simulink model "UAV_Research_Environment"  (R2025a)
settings: Solver=ode23t  StartTime=0.0  StopTime=130  MaxStep=2e-3  RelTol=1e-4  AbsTol=1e-3  EnableMultiTasking=on
InitFcn:
  | skipInitialization = false;
  | 
  | if evalin('base', ...
  |         'exist(''CONTROLLER_TUNING_ACTIVE'',''var'')')
  | 
  |     skipInitialization = evalin('base', ...
  |         'logical(CONTROLLER_TUNING_ACTIVE)');
  | end
  | 
  | if ~skipInitialization
  | 
  |     icraControllerPrepared = false;
  | 
  |     hasICRAVariables = evalin('base', ...
  |         ['exist(''AUTOPILOT'',''var'') && ' ...
  |          'exist(''ICRA_ACTIVE_CONTROLLER'',''var'') && ' ...
  |          'exist(''ICRA_ACTIVE_RUN_ID'',''var'')']);
  | 
  |     if hasICRAVariables
  | 
  |         icraControllerPrepared = evalin('base', ...
  |             ['isstruct(AUTOPILOT) && ' ...
  |              'isfield(AUTOPILOT,''info'') && ' ...
  |              'isfield(AUTOPILOT.info,''ICRAControllerID'') && ' ...
  |              'strcmp(string(AUTOPILOT.info.ICRAControllerID), ' ...
  |                     'string(ICRA_ACTIVE_CONTROLLER))']);
  | 
  |     end
  | 
  |     if icraControllerPrepared
  |         skipInitialization = true;
  |     end
  | end
  | 
  | if ~skipInitialization
  | 
  |     mdl = bdroot;
  | 
  |     mdl_file = get_param(mdl, 'FileName');
  | 
  |     project_root = fileparts(mdl_file);
  | 
  |     init_file = fullfile(project_root, 'initialize_project.m');
  | 
  |     if exist(init_file, 'file')
  | 
  |         run(init_file);
  | 
  |     else
  | 
  |         error('initialize_project.m was not found in the model folder.');
  | 
  |     end
  | end
values from neighbouring files (symbols this model uses):
  A_UAV = struct()    [UAV_analytical.m]
  AUTOPILOT = struct()    [UAV_autopilot.m]
  B_UAV = struct()    [UAV_block.m]
  D = A_UAV.source.propeller_diameter_m    [UAV_analytical.m]    (also in plot_controller_results.m = permute(                  D,                  order); plot_estimator_results.m = permute(              D,              order); plot_mission_results.m = permute(                  D,                  order); plot_touchdown_diagnostics.m = permute(                  D,                  order))
  OPERATOR_MODE = OPERATOR_MODE_MANUAL    [initialize_project.m]    (also in uav_remote_gui.m = uint8(0))
  P_ENV = struct()    [Environment.m]
  P_UAV = struct()    [UAV_simscape.m]
  s = sin(angle)    [uav_remote_gui.m]
  SENSOR = struct()    [UAV_sensors.m]
  TRAJECTORY_CONFIG = struct()    [UAV_trajectories.m]
  TRAJECTORY_ID = uint8(          trajectoryIDNumeric)    [UAV_trajectories.m]
  X = reshape(                  D,                  nt,                  [])    [plot_controller_results.m]    (also in plot_estimator_results.m = reshape(              D,              nt,              []); plot_mission_results.m; plot_touchdown_diagnostics.m; plot_trajectory_3d.m)
  Y = absolutePlanNED(1,:)    [plot_trajectory_3d.m]    (also in uav_remote_gui.m = positionNED(:,1))
  Z = landedCGDown -          absolutePlanNED(3,:)    [plot_trajectory_3d.m]    (also in uav_remote_gui.m = landedCGDown-positionNED(:,3))
undefined symbols (not defined in the file or in its folder): Acceleration_ref, F, fractalcoef, Light, MIL, Position_ref, Velocity_ref, Yaw_ref, YawRate_ref
libraries: sm_lib x49, nesl_utility x29, fl_lib x17, slpidlib x16, simulink x14, ee_lib x5, sdl_lib x4, aerolibwind2 x3, aerolibatmos2 x2, sensorbarometerlib x1, sensorgpslib x1, mspsensorlib x1
(part 2 of 9)

== system UAV_Research_Environment/Remote Controller/Automatic Operator ==
  Automatic Protocol : MATLAB Function  TreatAsAtomicUnit=on
  Protocol Table : Constant  Value=|  OutDataTypeStr=double
      | [AUTO_PROTOCOL.selected.armTime_s;
      |  AUTO_PROTOCOL.selected.runTime_s;
      |  AUTO_PROTOCOL.selected.disarmTime_s;
      |  AUTO_PROTOCOL.selected.stopTime_s]
  Simulation Time : Clock
  Trajectory ID : Constant  Value=TRAJECTORY_ID  OutDataTypeStr=uint8
  ArmCommand : Outport
  RunTrajectoryRequestID : Outport  Port=2
  wires:
  Simulation Time/1 -> Automatic Protocol/1(t)
  Trajectory ID/1 -> Automatic Protocol/2(TrajectoryID)
  Protocol Table/1 -> Automatic Protocol/3(ProtocolTable_s)
  Automatic Protocol/1(ArmCommand) -> ArmCommand/1
  Automatic Protocol/2(RunTrajectoryRequestID) -> RunTrajectoryRequestID/1

== system UAV_Research_Environment/Sensor/Barometer ==
  Env : Inport
  Barometer Sensor : sensorbarometerlib/Barometer  ConstantBias=SENSOR.Barometer.constantBias_Pa  NoiseDensity=SENSOR.Barometer.noiseDensity_Pa_sqrtHz  BiasInstability=SENSOR.Barometer.biasInstability_Pa  DecayFactor=SENSOR.Barometer.decayFactor  SeedDouble=SENSOR.Barometer.seed  SimulateUsing=Code generation
      settings: LibrarySourceBlock=uavsimlib/Barometer
  Bus Creator : BusCreator  Inputs=2
  Bus Selector : BusSelector  OutputSignals=Atmosphere.AirPressure
  Pressure Altitude Sensor : aerolibatmos2/Pressure Altitude  units=Metric (MKS)  action=Warning
  Zero-Order Hold : ZeroOrderHold  SampleTime=SENSOR.Barometer.sampleTime_s
  Barometer : Outport
  wires:
  Env/1 -> Bus Selector/1
  Bus Selector/1 -> Zero-Order Hold/1  "<AirPressure>"
  Zero-Order Hold/1 -> Barometer Sensor/1
  Barometer Sensor/1 -> Pressure Altitude Sensor/1, Bus Creator/1  "Pressure"
  Pressure Altitude Sensor/1 -> Bus Creator/2  "Altitude"
  Bus Creator/1 -> Barometer/1

== system UAV_Research_Environment/Sensor/GPS ==
  States : Inport
  Bus Creator : BusCreator  Inputs=2
  Bus Selector : BusSelector  OutputSignals=Position,Velocity
  GPS Sensor : sensorgpslib/GPS  DispRefFrame=NED  PositionInputFormat=Local  ReferenceLocation=SENSOR.GPS.referenceLocation_lla_deg_m  HorizontalPositionAccuracy=SENSOR.GPS.horizontalPositionAccuracy_m  VerticalPositionAccuracy=SENSOR.GPS.verticalPositionAccuracy_m  VelocityAccuracy=SENSOR.GPS.velocityAccuracy_m_s  DecayFactor=SENSOR.GPS.decayFactor  SeedDouble=SENSOR.GPS.seed  SimulateUsing=Code generation
      settings: LibrarySourceBlock=mspsensorlib/GPS
  Reshape : Reshape  OutputDimensionality=Row vector (2-D)
  Reshape1 : Reshape  OutputDimensionality=Row vector (2-D)
  Terminator : Terminator
  Terminator1 : Terminator
  Transpose2 : Math  Operator=transpose
  Transpose3 : Math  Operator=transpose
  Zero-Order Hold : ZeroOrderHold  SampleTime=SENSOR.GPS.sampleTime_s
  Zero-Order Hold1 : ZeroOrderHold  SampleTime=SENSOR.GPS.sampleTime_s
  GPS : Outport
  wires:
  States/1 -> Bus Selector/1
  Bus Selector/1 -> Zero-Order Hold/1  "<Position>"
  Bus Selector/2 -> Zero-Order Hold1/1  "<Velocity>"
  Zero-Order Hold1/1 -> Reshape1/1
  Zero-Order Hold/1 -> Reshape/1
  GPS Sensor/1 -> Transpose2/1  "LLA"
  GPS Sensor/2 -> Transpose3/1  "Velocity"
  Bus Creator/1 -> GPS/1
  Reshape/1 -> GPS Sensor/1
  Reshape1/1 -> GPS Sensor/2
  Transpose2/1 -> Bus Creator/1  "LLA"
  Transpose3/1 -> Bus Creator/2  "Velocity"
  GPS Sensor/3 -> Terminator/1
  GPS Sensor/4 -> Terminator1/1

== system UAV_Research_Environment/Sensor/IMU ==
  States : Inport
  Bus Creator : BusCreator  Inputs=2
  Bus Selector : BusSelector  OutputSignals=Acceleration,AngularRate,Attitude.Q
  IMU Sensor : mspsensorlib/IMU  DispRefFrame=NED  TemperaturePort=off  Temperature=SENSOR.IMU.temperature_C  MagneticFieldPort=off  MagneticFieldNED=SENSOR.IMU.mag.fieldNED_uT  MagneticFieldENU=[ -2.4169, 27.5550, 16.0849 ]  SeedDouble=SENSOR.IMU.seed  SimulateUsing=Code generation  AccelParamsMeasurementRange=SENSOR.IMU.accel.maximumReading_m_s2  AccelParamsResolution=SENSOR.IMU.accel.resolution_m_s2_LSB  AccelParamsConstantBias=SENSOR.IMU.accel.constantBias_m_s2  AccelParamsAxesMisalignment=SENSOR.IMU.accel.axesSkew_percent  AccelParamsNoiseDensity=SENSOR.IMU.accel.velocityRandomWalk_m_s2_sqrtHz  AccelParamsBiasInstability=SENSOR.IMU.accel.biasInstability_m_s2  AccelParamsBiasInstabilityNumerator=fractalcoef().Numerator  AccelParamsBiasInstabilityDenominator=fractalcoef().Denominator  AccelParamsRandomWalk=SENSOR.IMU.accel.accelerationRandomWalk_m_s2_sqrtHz  AccelParamsNoiseType=double-sided  AccelParamsTemperatureBias=[ 0, 0, 0 ]  AccelParamsTemperatureScaleFactor=[ 0, 0, 0 ]  GyroParamsMeasurementRange=SENSOR.IMU.gyro.maximumReading_rad_s  GyroParamsResolution=SENSOR.IMU.gyro.resolution_rad_s_LSB  GyroParamsConstantBias=SENSOR.IMU.gyro.constantBias_rad_s  GyroParamsAxesMisalignment=SENSOR.IMU.gyro.axesSkew_percent  GyroParamsAccelerationBias=SENSOR.IMU.gyro.biasFromAcceleration_rad_s_per_m_s2  GyroParamsNoiseDensity=SENSOR.IMU.gyro.angleRandomWalk_rad_s_sqrtHz  GyroParamsBiasInstability=SENSOR.IMU.gyro.biasInstability_rad_s  GyroParamsBiasInstabilityNumerator=fractalcoef().Numerator  GyroParamsBiasInstabilityDenominator=fractalcoef().Denominator  GyroParamsRandomWalk=SENSOR.IMU.gyro.rateRandomWalk_rad_s_sqrtHz  GyroParamsNoiseType=double-sided  GyroParamsTemperatureBias=SENSOR.IMU.gyro.temperatureBias_rad_s_per_C  GyroParamsTemperatureScaleFactor=SENSOR.IMU.gyro.temperatureScaleFactor_percent_per_C  MagParamsMeasurementRange=SENSOR.IMU.mag.maximumReading_uT  MagParamsResolution=SENSOR.IMU.mag.resolution_uT_LSB  MagParamsConstantBias=SENSOR.IMU.mag.constantBias_uT  MagParamsAxesMisalignment=SENSOR.IMU.mag.axesSkew_percent  MagParamsNoiseDensity=SENSOR.IMU.mag.whiteNoisePSD_uT_sqrtHz  MagParamsBiasInstability=SENSOR.IMU.mag.biasInstability_uT  MagParamsBiasInstabilityNumerator=fractalcoef().Numerator  MagParamsBiasInstabilityDenominator=fractalcoef().Denominator  MagParamsRandomWalk=SENSOR.IMU.mag.randomWalk_uT_sqrtHz  MagParamsNoiseType=double-sided  MagParamsTemperatureBias=SENSOR.IMU.mag.temperatureBias_uT_per_C  MagParamsTemperatureScaleFactor=SENSOR.IMU.mag.temperatureScaleFactor_percent_per_C
  Matrix Multiply : Product  Multiplication=Matrix(*)
  Quaternions to Direction Cosine Matrix : Quat2Dcm
  Reshape : Reshape  OutputDimensionality=Row vector (2-D)
  Reshape2 : Reshape  OutputDimensionality=Customize  OutputDimensions=[3 1]
  Transpose{,1,4..6} (5 alike) : Math  Operator=transpose
  Zero-Order Hold{,1..3} (4 alike) : ZeroOrderHold  SampleTime=SENSOR.IMU.sampleTime_s
  IMU : Outport
  MagneticField : Outport  Port=2
  wires:
  States/1 -> Bus Selector/1
  Bus Selector/1 -> Zero-Order Hold/1  "<Acceleration>"
  Bus Selector/3 -> Quaternions to Direction Cosine Matrix/1  "<Q>"
  Quaternions to Direction Cosine Matrix/1 -> Transpose/1, Zero-Order Hold2/1
  Bus Selector/2 -> Zero-Order Hold3/1  "<AngularRate>"
  Matrix Multiply/1 -> Zero-Order Hold1/1  "Omega_ned"
  IMU Sensor/1 -> Transpose4/1  "Accel"
  IMU Sensor/2 -> Transpose5/1  "Gyro"
  Bus Creator/1 -> IMU/1
  Zero-Order Hold/1 -> Reshape/1
  IMU Sensor/3 -> Transpose6/1
  Reshape/1 -> IMU Sensor/1
  Zero-Order Hold1/1 -> Transpose1/1
  Transpose4/1 -> Bus Creator/1  "Accel"
  Transpose5/1 -> Bus Creator/2  "Gyro"
  Transpose6/1 -> MagneticField/1
  Reshape2/1 -> Matrix Multiply/2
  Zero-Order Hold2/1 -> IMU Sensor/3
  Transpose/1 -> Matrix Multiply/1  "DCM_eb"
  Zero-Order Hold3/1 -> Reshape2/1
  Transpose1/1 -> IMU Sensor/2

== system UAV_Research_Environment/Sensor/Magnetometer ==
  MagneticField : Inport
  Bus Creator : BusCreator  Inputs=1
  Magnetometer : Outport
  wires:
  MagneticField/1 -> Bus Creator/1  "MagneticField"
  Bus Creator/1 -> Magnetometer/1

== system UAV_Research_Environment/UAV Plant/UAV Analytical [ODEs] ==
  Omega : Inport  PortDimensions=[4 1]
  Env : Inport  Port=2
  Attitude Kinematics : Subsystem
      settings: PortSchema="{\"entries\":[{\"content\":{\"sides\":[{\"content\":{\"connectorIds\":[\"Out3\"]},\"type\":\"ConnectorPlacement.EquallySpacedRectSide\",\"uuid\":\"9dff6125-8704-4564-9479-4179f05149c8\"},{\"content\":{\"connectorIds\":[\"Out1\",\"Out2\"],\"side\":\"RIGHT\"},\"type\":\"ConnectorPlacement.EquallySpacedRectSide\",\"uuid\":\"bf94854b-7c24-453f-8a34-028b591b285b\"},{\"content\":{\"side\":\"TOP\"},\"type\":\"ConnectorPlacement.EquallySpacedRectSide\",\"uuid\":\"13a26fb3-0875-4110-aca8-48b2789d508d\"},{\"content\":{\"connectorIds\":[\"In1\"],\"side\":\"BOTTOM\"},\"type\":\"ConnectorPlacement.EquallySpacedRectSide\",\"uuid\":\"645477ff-464b-45b4-8561-14b6e33c2c53\"}]},\"type\":\"ConnectorPlacement.EquallySpacedConnector\",\"uuid\":\"ec2d45a2-6558-4c38-a80a-f2c514fd0af7\"}],\"packageUris\":[\"http://schema.mathworks.com/mf0/Connector/R2020b\"],\"version\":\"1.0\"}"
  Bus Selector : BusSelector  OutputSignals=Gravity,Wind.v,Atmosphere.AirDensity,Wind.w
  Ground Contact : Subsystem
  Mux : Mux  Inputs=3
  Pitch Moment : Subsystem
  Roll Moment : Subsystem
  Rotational Dynamics : Subsystem
      settings: PortSchema="{\"entries\":[{\"content\":{\"sides\":[{\"content\":{\"connectorIds\":[\"In1\",\"In2\"]},\"type\":\"ConnectorPlacement.EquallySpacedRectSide\",\"uuid\":\"b3993310-afcd-4214-b563-33689f9bf855\"},{\"content\":{\"side\":\"RIGHT\"},\"type\":\"ConnectorPlacement.EquallySpacedRectSide\",\"uuid\":\"528b295d-3dab-4a73-9569-b357e78729a6\"},{\"content\":{\"connectorIds\":[\"Out1\"],\"side\":\"TOP\"},\"type\":\"ConnectorPlacement.EquallySpacedRectSide\",\"uuid\":\"2fd251fa-5731-4e9d-a8cb-8d2c450fe105\"},{\"content\":{\"side\":\"BOTTOM\"},\"type\":\"ConnectorPlacement.EquallySpacedRectSide\",\"uuid\":\"3d992d66-ff37-470d-9d82-4b7598c36df4\"}]},\"type\":\"ConnectorPlacement.EquallySpacedConnector\",\"uuid\":\"9bc87e62-5e61-4b2d-bc0c-f9f90b87fbd3\"}],\"packageUris\":[\"http://schema.mathworks.com/mf0/Connector/R2020b\"],\"version\":\"1.0\"}"
  Rotor Force : Subsystem
  Rotor Reaction Torque : Subsystem
  Rotor Thrust : Subsystem
  State Outputs : Subsystem
  Sum : Sum  Inputs=|++
  Sum1 : Sum  Inputs=|++
  Translational Dynamics : Subsystem
      settings: PortSchema="{\"entries\":[{\"content\":{\"sides\":[{\"content\":{\"connectorIds\":[\"In1\",\"In2\"]},\"type\":\"ConnectorPlacement.EquallySpacedRectSide\",\"uuid\":\"e7713371-9d44-4df7-ad98-126530e47f57\"},{\"content\":{\"connectorIds\":[\"Out1\",\"Out2\",\"Out3\"],\"side\":\"RIGHT\"},\"type\":\"ConnectorPlacement.EquallySpacedRectSide\",\"uuid\":\"b198966c-7c08-4a9a-99fe-2713033265e1\"},{\"content\":{\"connectorIds\":[\"In3\",\"In4\",\"In5\"],\"side\":\"TOP\"},\"type\":\"ConnectorPlacement.EquallySpacedRectSide\",\"uuid\":\"dc79653a-0d9e-4550-92f6-01194e9ba711\"}]},\"type\":\"ConnectorPlacement.EquallySpacedConnector\",\"uuid\":\"db8e1ac8-22bc-47be-9eb6-51b7df091317\"}],\"packageUris\":[\"http://schema.mathworks.com/mf0/Connector/R2020b\"],\"version\":\"1.0\"}"
  Yaw Moment : Subsystem
  States : Outport
  wires:
  Omega/1 -> Rotor Reaction Torque/1(Omega), Rotor Thrust/1(Omega)
  Rotor Thrust/1(T) -> Rotor Force/1(T), Roll Moment/1(T), Pitch Moment/1(T)
  Rotor Reaction Torque/1(Q) -> Yaw Moment/1(Q)
  Pitch Moment/1(Tau_y) -> Mux/2
  Roll Moment/1(Tau_x) -> Mux/1
  Yaw Moment/1(Tau_z) -> Mux/3
  Mux/1 -> Sum1/1  "Tau_body"
  Rotor Force/1(F_body) -> Sum/1
  Rotational Dynamics/1(Omega_body) -> State Outputs/6(Omega_body), Attitude Kinematics/1(Omega_body), Ground Contact/4(Omega_body)
  Attitude Kinematics/3(R_BN) -> Ground Contact/3(R_BN), Translational Dynamics/2(R_BN)
  Attitude Kinematics/1(Euler) -> State Outputs/4(Euler)
  Translational Dynamics/1(v_ned) -> Ground Contact/2(v_ned), State Outputs/1(v_ned)
  Translational Dynamics/2(p_ned) -> Ground Contact/1(p_ned), State Outputs/2(p_ned)
  State Outputs/1(States) -> States/1
  Env/1 -> Bus Selector/1
  Bus Selector/1 -> Translational Dynamics/5(g)  "<Gravity>"
  Bus Selector/2 -> Translational Dynamics/4(Wind_v)  "<v>"
  Bus Selector/3 -> Translational Dynamics/3(rho)  "<AirDensity>"
  Bus Selector/4 -> Rotational Dynamics/2(Wind_w)  "<w>"
  Translational Dynamics/3(a_ned) -> State Outputs/3(a_ned)
  Attitude Kinematics/2(Q) -> State Outputs/5(Q)
  Sum/1 -> Translational Dynamics/1(F_body)
  Ground Contact/1(F_ground_body) -> Sum/2
  Sum1/1 -> Rotational Dynamics/1("Tau_body ")
  Ground Contact/2(Tau_ground_body) -> Sum1/2

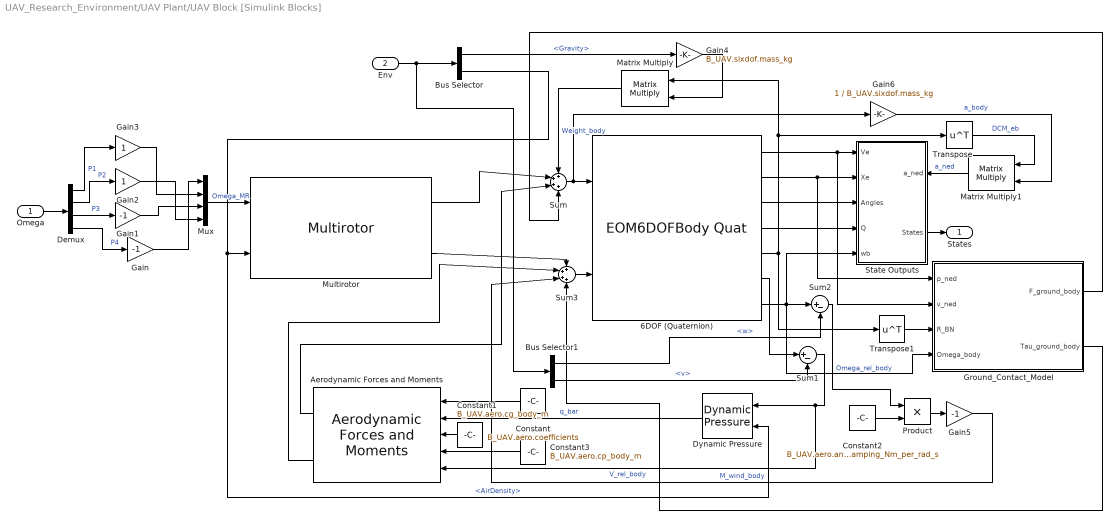
== system UAV_Research_Environment/UAV Plant/UAV Block [Simulink Blocks] ==
  Omega : Inport  PortDimensions=[4 1]
  Env : Inport  Port=2
  6DOF (Quaternion) : EOM6DOFBodyQuat  xme_0=B_UAV.sixdof.initial_position_ned_m'  Vm_0=B_UAV.sixdof.initial_velocity_body_m_s'  eul_0=B_UAV.sixdof.initial_euler_rad'  pm_0=B_UAV.sixdof.initial_body_rates_rad_s'  mass_0=B_UAV.sixdof.mass_kg  inertia=B_UAV.sixdof.inertia_kgm2
  "Aerodynamic Forces and Moments  " : aerolibadyn/Aerodynamic Forces and Moments   inputAxes=Wind  outputForceAxes=Body  outputMomentAxes=Body  S=B_UAV.aero.reference_area_m2  b=B_UAV.aero.reference_span_m  cbar=B_UAV.aero.reference_length_m
  Bus Selector : BusSelector  OutputSignals=Gravity,Atmosphere.AirDensity
  Bus Selector1 : BusSelector  OutputSignals=Wind.w,Wind.v
  Constant : Constant  Value=B_UAV.aero.coefficients
  Constant1 : Constant  Value=B_UAV.aero.cg_body_m
  Constant2 : Constant  Value=B_UAV.aero.angular_damping_Nm_per_rad_s
  Constant3 : Constant  Value=B_UAV.aero.cp_body_m
  Demux : Demux
  Dynamic Pressure : aerolibasang/Dynamic Pressure
  Gain : Gain  Gain=-1
  Gain1 : Gain  Gain=-1
  Gain2 : Gain
  Gain3 : Gain
  Gain4 : Gain  Gain=B_UAV.sixdof.mass_kg
  Gain5 : Gain  Gain=-1
  Gain6 : Gain  Gain=1 / B_UAV.sixdof.mass_kg
  Ground_Contact_Model : MATLAB Function  TreatAsAtomicUnit=on
  Matrix Multiply : Product  Multiplication=Matrix(*)
  Matrix Multiply1 : Product  Multiplication=Matrix(*)
  Multirotor : Multirotor  armLength=B_UAV.multirotor.arm_length_m  rotorHeight=B_UAV.multirotor.rotor_height_m  CT=B_UAV.multirotor.CT  CQ=B_UAV.multirotor.CQ  radius=B_UAV.multirotor.radius_m
  Mux : Mux
  Product : Product
  State Outputs : Subsystem
      settings: PortSchema="{\"entries\":[{\"content\":{\"sides\":[{\"content\":{\"connectorIds\":[\"In1\",\"In2\",\"In3\",\"In4\",\"In5\"]},\"type\":\"ConnectorPlacement.EquallySpacedRectSide\",\"uuid\":\"f801e9e4-3e2d-4270-9414-2c8f22496f29\"},{\"content\":{\"connectorIds\":[\"In6\",\"Out1\"],\"side\":\"RIGHT\"},\"type\":\"ConnectorPlacement.EquallySpacedRectSide\",\"uuid\":\"c825f747-4acf-4485-a014-2278f8856f7a\"},{\"content\":{\"side\":\"TOP\"},\"type\":\"ConnectorPlacement.EquallySpacedRectSide\",\"uuid\":\"300a9a75-5249-49f1-bbea-59b79bcae31d\"}]},\"type\":\"ConnectorPlacement.EquallySpacedConnector\",\"uuid\":\"82c663c5-bb4d-48ca-be4c-f6c508d5737f\"}],\"packageUris\":[\"http://schema.mathworks.com/mf0/Connector/R2020b\"],\"version\":\"1.0\"}"
  Sum : Sum  Inputs=++++
  Sum1 : Sum  Inputs=|+-
  Sum2 : Sum  Inputs=|+-
  Sum3 : Sum  Inputs=++++
  Transpose : Math  Operator=transpose
  Transpose1 : Math  Operator=transpose
  States : Outport
  wires:
  Omega/1 -> Demux/1
  Demux/1 -> Gain3/1  "P1"
  Demux/2 -> Gain2/1  "P2"
  Demux/3 -> Gain1/1  "P3"
  Demux/4 -> Gain/1  "P4"
  Mux/1 -> Multirotor/1  "Omega_MR"
  Gain/1 -> Mux/1
  Gain3/1 -> Mux/2
  Gain1/1 -> Mux/3
  Gain2/1 -> Mux/4
  Gain4/1 -> Matrix Multiply/2
  6DOF (Quaternion)/5 -> Transpose1/1, Transpose/1, Matrix Multiply/1
  Matrix Multiply/1 -> Sum/1  "Weight_body"
  Sum/1 -> Gain6/1, 6DOF (Quaternion)/1
  Multirotor/1 -> Sum/2
  6DOF (Quaternion)/1 -> Ground_Contact_Model/2(v_ned), State Outputs/1(Ve)
  6DOF (Quaternion)/2 -> Ground_Contact_Model/1(p_ned), State Outputs/2(Xe)
  6DOF (Quaternion)/3 -> State Outputs/3(Angles)
  6DOF (Quaternion)/4 -> State Outputs/4(Q)
  State Outputs/1(States) -> States/1
  Bus Selector/1 -> Gain4/1  "<Gravity>"
  Bus Selector/2 -> Multirotor/2, Dynamic Pressure/2  "<AirDensity>"
  Env/1 -> Bus Selector/1, Bus Selector1/1
  Bus Selector1/1 -> Sum2/2  "<w>"
  Bus Selector1/2 -> Sum1/2  "<v>"
  6DOF (Quaternion)/6 -> Sum1/1
  Sum1/1 -> "Aerodynamic Forces and Moments  "/5, Dynamic Pressure/1  "V_rel_body"
  6DOF (Quaternion)/7 -> Sum2/1, State Outputs/5(wb), Ground_Contact_Model/4(Omega_body)
  Sum2/1 -> Product/1  "Omega_rel_body"
  Dynamic Pressure/1 -> "Aerodynamic Forces and Moments  "/2  "q_bar"
  Constant/1 -> "Aerodynamic Forces and Moments  "/1
  Constant1/1 -> "Aerodynamic Forces and Moments  "/3
  "Aerodynamic Forces and Moments  "/1 -> Sum/3
  Sum3/1 -> 6DOF (Quaternion)/2
  Multirotor/2 -> Sum3/1
  "Aerodynamic Forces and Moments  "/2 -> Sum3/2
  Constant2/1 -> Product/2
  Product/1 -> Gain5/1
  Gain5/1 -> Sum3/3  "M_wind_body"
  Constant3/1 -> "Aerodynamic Forces and Moments  "/4
  Gain6/1 -> Matrix Multiply1/2  "a_body"
  Transpose/1 -> Matrix Multiply1/1  "DCM_eb"
  Matrix Multiply1/1 -> State Outputs/6(a_ned)  "a_ned"
  Ground_Contact_Model/1(F_ground_body) -> Sum/4
  Ground_Contact_Model/2(Tau_ground_body) -> Sum3/4
  Transpose1/1 -> Ground_Contact_Model/3(R_BN)

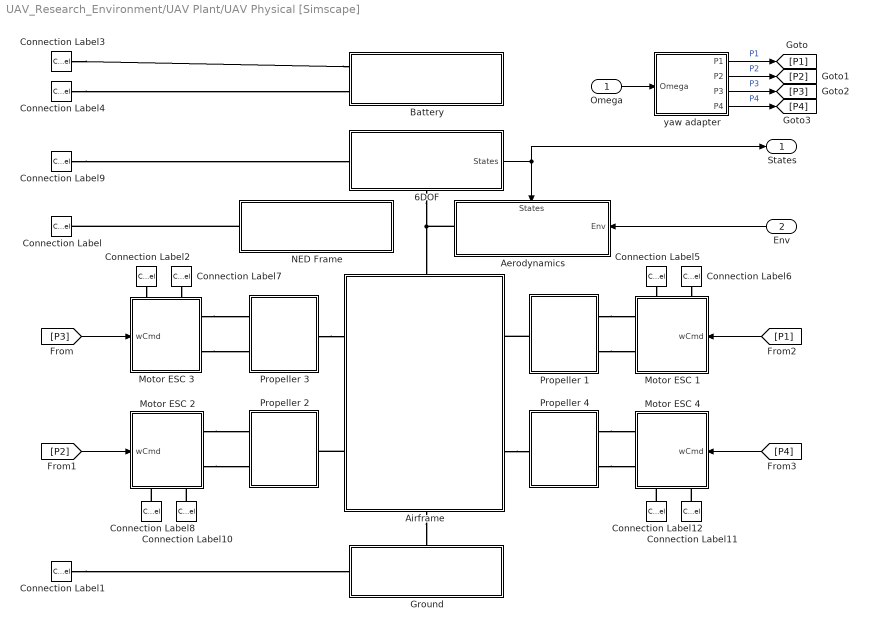
== system UAV_Research_Environment/UAV Plant/UAV Physical [Simscape] ==
  Omega : Inport  PortDimensions=[4 1]
  Env : Inport  Port=2
  6DOF : Subsystem
      settings: PortSchema="{\"entries\":[{\"content\":{\"sides\":[{\"content\":{\"connectorIds\":[\"LConn1\"]},\"type\":\"ConnectorPlacement.EquallySpacedRectSide\",\"uuid\":\"e25d5fac-f14f-4db4-ba7c-0db3b640b000\"},{\"content\":{\"connectorIds\":[\"Out1\"],\"side\":\"RIGHT\"},\"type\":\"ConnectorPlacement.EquallySpacedRectSide\",\"uuid\":\"ece4c34b-2450-4f31-b634-0268ecd3db77\"},{\"content\":{\"side\":\"TOP\"},\"type\":\"ConnectorPlacement.EquallySpacedRectSide\",\"uuid\":\"45ba64a1-5c3e-41bf-9d86-ff80caef146a\"},{\"content\":{\"connectorIds\":[\"RConn1\"],\"side\":\"BOTTOM\"},\"type\":\"ConnectorPlacement.EquallySpacedRectSide\",\"uuid\":\"5fe681e2-89b9-4752-a871-8a0d7d1f1229\"}]},\"type\":\"ConnectorPlacement.EquallySpacedConnector\",\"uuid\":\"3dfbf8ce-831d-48fb-8ef5-da555b42ce83\"}],\"packageUris\":[\"http://schema.mathworks.com/mf0/Connector/R2020b\"],\"version\":\"1.0\"}"
  Aerodynamics : Subsystem
      settings: PortSchema="{\"entries\":[{\"content\":{\"sides\":[{\"content\":{\"connectorIds\":[\"LConn1\"]},\"type\":\"ConnectorPlacement.EquallySpacedRectSide\",\"uuid\":\"ccbff83c-f4a8-47eb-bbec-6359b61a398f\"},{\"content\":{\"connectorIds\":[\"In2\"],\"side\":\"RIGHT\"},\"type\":\"ConnectorPlacement.EquallySpacedRectSide\",\"uuid\":\"cdd614a3-a500-4946-a9f7-466a70707194\"},{\"content\":{\"connectorIds\":[\"In1\"],\"side\":\"TOP\"},\"type\":\"ConnectorPlacement.EquallySpacedRectSide\",\"uuid\":\"6b69b0d1-68de-4a3a-8405-962f6025eb08\"}]},\"type\":\"ConnectorPlacement.EquallySpacedConnector\",\"uuid\":\"9c7a8fe4-8ea8-4366-82cf-150671760d77\"}],\"packageUris\":[\"http://schema.mathworks.com/mf0/Connector/R2020b\"],\"version\":\"1.0\"}"
  Airframe : Subsystem
      settings: PortSchema="{\"entries\":[{\"content\":{\"sides\":[{\"content\":{\"connectorIds\":[\"LConn1\",\"LConn2\"]},\"type\":\"ConnectorPlacement.EquallySpacedRectSide\",\"uuid\":\"7cba0a73-b9eb-47c6-b800-fc4f8e3dfd2f\"},{\"content\":{\"connectorIds\":[\"RConn1\",\"RConn2\"],\"side\":\"RIGHT\"},\"type\":\"ConnectorPlacement.EquallySpacedRectSide\",\"uuid\":\"fa446dff-d878-436a-aac5-559c768d81f7\"},{\"content\":{\"connectorIds\":[\"LConn3\"],\"side\":\"TOP\"},\"type\":\"ConnectorPlacement.EquallySpacedRectSide\",\"uuid\":\"74e12617-ead0-48ff-8362-b73d9a2be5cd\"},{\"content\":{\"connectorIds\":[\"RConn3\"],\"side\":\"BOTTOM\"},\"type\":\"ConnectorPlacement.EquallySpacedRectSide\",\"uuid\":\"e22a0e6f-9b52-4c3c-a523-f720ff46fe61\"}]},\"type\":\"ConnectorPlacement.EquallySpacedConnector\",\"uuid\":\"27fc30b3-6c35-43ed-8881-9207c20b6357\"}],\"packageUris\":[\"http://schema.mathworks.com/mf0/Connector/R2020b\"],\"version\":\"1.0\"}"
  Battery : Subsystem
  Connection Label : ConnectionLabel  Label=NED
  Connection Label1 : ConnectionLabel  Label=NED
  Connection Label{3,6..7,10..11} (5 alike) : ConnectionLabel  Label=VCC
  Connection Label{2,4..5,8,12} (5 alike) : ConnectionLabel  Label=GND
  Connection Label9 : ConnectionLabel  Label=NED
  Ground : Subsystem
      settings: PortSchema="{\"entries\":[{\"content\":{\"sides\":[{\"content\":{\"connectorIds\":[\"LConn1\"]},\"type\":\"ConnectorPlacement.EquallySpacedRectSide\",\"uuid\":\"df27cac0-d486-4fe7-a24b-0ab0296c81c9\"},{\"content\":{\"side\":\"RIGHT\"},\"type\":\"ConnectorPlacement.EquallySpacedRectSide\",\"uuid\":\"7e7f7d4d-0e7a-4771-811c-9aec9b97b2c8\"},{\"content\":{\"connectorIds\":[\"LConn2\"],\"side\":\"TOP\"},\"type\":\"ConnectorPlacement.EquallySpacedRectSide\",\"uuid\":\"6525dab8-ce29-449f-bd79-e0f9e77d4aa7\"}]},\"type\":\"ConnectorPlacement.EquallySpacedConnector\",\"uuid\":\"5c96d7c2-b260-47d1-9ef2-16cc4cd02942\"}],\"packageUris\":[\"http://schema.mathworks.com/mf0/Connector/R2020b\"],\"version\":\"1.0\"}"
  Motor ESC 1 : Subsystem
      settings: PortSchema="{\"entries\":[{\"content\":{\"sides\":[{\"content\":{\"connectorIds\":[\"LConn1\",\"LConn2\"]},\"type\":\"ConnectorPlacement.EquallySpacedRectSide\",\"uuid\":\"71a7681e-d316-41c3-8134-2ee0309c2707\"},{\"content\":{\"connectorIds\":[\"In1\"],\"side\":\"RIGHT\"},\"type\":\"ConnectorPlacement.EquallySpacedRectSide\",\"uuid\":\"90d7ee2b-0fce-46ec-a51b-0232e8fd2cbc\"},{\"content\":{\"connectorIds\":[\"LConn3\",\"LConn4\"],\"side\":\"TOP\"},\"type\":\"ConnectorPlacement.EquallySpacedRectSide\",\"uuid\":\"1e39919d-7cbd-4646-a3ea-c7d65814bae6\"},{\"content\":{\"side\":\"BOTTOM\"},\"type\":\"ConnectorPlacement.EquallySpacedRectSide\",\"uuid\":\"a2c9eda9-e0f5-43e3-b591-1a9dcc93eb0e\"}]},\"type\":\"ConnectorPlacement.EquallySpacedConnector\",\"uuid\":\"c047d66f-8d7d-4abc-9544-94bba003335f\"}],\"packageUris\":[\"http://schema.mathworks.com/mf0/Connector/R2020b\"],\"version\":\"1.0\"}"
  Motor ESC 2 : Subsystem
      settings: PortSchema="{\"entries\":[{\"content\":{\"sides\":[{\"content\":{\"connectorIds\":[\"LConn1\",\"LConn2\"]},\"type\":\"ConnectorPlacement.EquallySpacedRectSide\",\"uuid\":\"71a7681e-d316-41c3-8134-2ee0309c2707\"},{\"content\":{\"connectorIds\":[\"In1\"],\"side\":\"RIGHT\"},\"type\":\"ConnectorPlacement.EquallySpacedRectSide\",\"uuid\":\"90d7ee2b-0fce-46ec-a51b-0232e8fd2cbc\"},{\"content\":{\"side\":\"TOP\"},\"type\":\"ConnectorPlacement.EquallySpacedRectSide\",\"uuid\":\"1e39919d-7cbd-4646-a3ea-c7d65814bae6\"},{\"content\":{\"connectorIds\":[\"RConn1\",\"RConn2\"],\"side\":\"BOTTOM\"},\"type\":\"ConnectorPlacement.EquallySpacedRectSide\",\"uuid\":\"a2c9eda9-e0f5-43e3-b591-1a9dcc93eb0e\"}]},\"type\":\"ConnectorPlacement.EquallySpacedConnector\",\"uuid\":\"c047d66f-8d7d-4abc-9544-94bba003335f\"}],\"packageUris\":[\"http://schema.mathworks.com/mf0/Connector/R2020b\"],\"version\":\"1.0\"}"
  Motor ESC 3 : Subsystem
      settings: PortSchema="{\"entries\":[{\"content\":{\"sides\":[{\"content\":{\"connectorIds\":[\"LConn1\",\"LConn2\"]},\"type\":\"ConnectorPlacement.EquallySpacedRectSide\",\"uuid\":\"71a7681e-d316-41c3-8134-2ee0309c2707\"},{\"content\":{\"connectorIds\":[\"In1\"],\"side\":\"RIGHT\"},\"type\":\"ConnectorPlacement.EquallySpacedRectSide\",\"uuid\":\"90d7ee2b-0fce-46ec-a51b-0232e8fd2cbc\"},{\"content\":{\"connectorIds\":[\"LConn3\",\"LConn4\"],\"side\":\"TOP\"},\"type\":\"ConnectorPlacement.EquallySpacedRectSide\",\"uuid\":\"1e39919d-7cbd-4646-a3ea-c7d65814bae6\"},{\"content\":{\"side\":\"BOTTOM\"},\"type\":\"ConnectorPlacement.EquallySpacedRectSide\",\"uuid\":\"a2c9eda9-e0f5-43e3-b591-1a9dcc93eb0e\"}]},\"type\":\"ConnectorPlacement.EquallySpacedConnector\",\"uuid\":\"c047d66f-8d7d-4abc-9544-94bba003335f\"}],\"packageUris\":[\"http://schema.mathworks.com/mf0/Connector/R2020b\"],\"version\":\"1.0\"}"
  Motor ESC 4 : Subsystem
      settings: PortSchema="{\"entries\":[{\"content\":{\"sides\":[{\"content\":{\"connectorIds\":[\"LConn1\",\"LConn2\"]},\"type\":\"ConnectorPlacement.EquallySpacedRectSide\",\"uuid\":\"71a7681e-d316-41c3-8134-2ee0309c2707\"},{\"content\":{\"connectorIds\":[\"In1\"],\"side\":\"RIGHT\"},\"type\":\"ConnectorPlacement.EquallySpacedRectSide\",\"uuid\":\"90d7ee2b-0fce-46ec-a51b-0232e8fd2cbc\"},{\"content\":{\"side\":\"TOP\"},\"type\":\"ConnectorPlacement.EquallySpacedRectSide\",\"uuid\":\"1e39919d-7cbd-4646-a3ea-c7d65814bae6\"},{\"content\":{\"connectorIds\":[\"RConn1\",\"RConn2\"],\"side\":\"BOTTOM\"},\"type\":\"ConnectorPlacement.EquallySpacedRectSide\",\"uuid\":\"a2c9eda9-e0f5-43e3-b591-1a9dcc93eb0e\"}]},\"type\":\"ConnectorPlacement.EquallySpacedConnector\",\"uuid\":\"c047d66f-8d7d-4abc-9544-94bba003335f\"}],\"packageUris\":[\"http://schema.mathworks.com/mf0/Connector/R2020b\"],\"version\":\"1.0\"}"
  NED Frame : Subsystem
  Propeller 1 : Subsystem
  Propeller 2 : Subsystem
  Propeller 3 : Subsystem
  Propeller 4 : Subsystem
  yaw adapter : MATLAB Function  TreatAsAtomicUnit=on
  States : Outport
  wires:
  6DOF/1(States) -> States/1, Aerodynamics/1(States)
  Env/1 -> Aerodynamics/2(Env)
  yaw adapter/1(P1) -> [P1]  "P1"
  yaw adapter/2(P2) -> [P2]  "P2"
  yaw adapter/3(P3) -> [P3]  "P3"
  yaw adapter/4(P4) -> [P4]  "P4"
  [P3] -> Motor ESC 3/1(wCmd)
  [P2] -> Motor ESC 2/1(wCmd)
  [P1] -> Motor ESC 1/1(wCmd)
  [P4] -> Motor ESC 4/1(wCmd)
  Omega/1 -> yaw adapter/1(Omega)
  connections:
  Propeller 1/LConn1 -- Airframe/RConn1
  NED Frame/LConn1 -- Connection Label/LConn1
  6DOF/RConn1 -- Aerodynamics/LConn1 -- Airframe/LConn3
  Connection Label1/LConn1 -- Ground/LConn1
  Propeller 3/LConn1 -- Airframe/LConn1
  Airframe/RConn3 -- Ground/LConn2
  Connection Label6/LConn1 -- Motor ESC 1/LConn4
  Motor ESC 3/LConn2 -- Propeller 3/RConn2
  Propeller 1/RConn2 -- Motor ESC 1/LConn2
  Propeller 1/RConn1 -- Motor ESC 1/LConn1
  Connection Label5/LConn1 -- Motor ESC 1/LConn3
  Airframe/LConn2 -- Propeller 2/LConn1
  Propeller 4/RConn1 -- Motor ESC 4/LConn1
  Propeller 4/RConn2 -- Motor ESC 4/LConn2
  Motor ESC 2/LConn1 -- Propeller 2/RConn1
  Motor ESC 2/LConn2 -- Propeller 2/RConn2
  Motor ESC 3/LConn1 -- Propeller 3/RConn1
  Connection Label4/LConn1 -- Battery/LConn2
  Connection Label9/LConn1 -- 6DOF/LConn1
  Connection Label7/LConn1 -- Motor ESC 3/LConn3
  Connection Label2/LConn1 -- Motor ESC 3/LConn4
  Connection Label8/LConn1 -- Motor ESC 2/RConn2
  Connection Label10/LConn1 -- Motor ESC 2/RConn1
  Connection Label11/LConn1 -- Motor ESC 4/RConn2
  Connection Label12/LConn1 -- Motor ESC 4/RConn1
  Connection Label3/LConn1 -- Battery/LConn1
  Airframe/RConn2 -- Propeller 4/LConn1

== system UAV_Research_Environment/Autopilot/Flight Control/Controller Supervisor ==
  FlightManagement : Inport
  "AND " : Logic  IconShape=distinctive  AllPortsSameDT=off  OutDataTypeStr=boolean
  Bus Creator : BusCreator  Inputs=2
  Bus Selector : BusSelector  OutputSignals=mode,armed,reset
  "Compare To Constant Trajectory " : simulink/Logic and Bit Operations/Compare To Constant  relop===  const=AUTOPILOT.mode.trajectory  OutDataTypeStr=boolean
  "Compare To Constant navFailsafe " : simulink/Logic and Bit Operations/Compare To Constant  relop===  const=AUTOPILOT.mode.navFailsafe  OutDataTypeStr=boolean
  Logical Operator : Logic  Operator=OR  AllPortsSameDT=off  OutDataTypeStr=boolean
  NOT : Logic  Operator=NOT  IconShape=distinctive  AllPortsSameDT=off  OutDataTypeStr=boolean
  "OR " : Logic  Operator=OR  IconShape=distinctive  AllPortsSameDT=off  OutDataTypeStr=boolean
  StateController : Outport
  wires:
  Bus Selector/3 -> "OR "/1  "<reset>"
  FlightManagement/1 -> Bus Selector/1
  Bus Selector/1 -> "Compare To Constant navFailsafe "/1, "Compare To Constant Trajectory "/1  "<mode>"
  Bus Selector/2 -> "AND "/2  "<armed>"
  NOT/1 -> "OR "/2
  "AND "/1 -> NOT/1, Bus Creator/1  "enableController"
  "OR "/1 -> Bus Creator/2  "resetController"
  Bus Creator/1 -> StateController/1
  "Compare To Constant navFailsafe "/1 -> Logical Operator/1
  "Compare To Constant Trajectory "/1 -> Logical Operator/2
  Logical Operator/1 -> "AND "/1

== system UAV_Research_Environment/Autopilot/Flight Control/Error Computation ==
  EstimatedStates : Inport
  Reference : Inport  Port=2
  Bus Creator : BusCreator  Inputs=2
  Bus Selector1 : BusSelector  OutputSignals=Position_ref,Yaw_ref
  Bus Selector2 : BusSelector  OutputSignals=Position,Attitude.Euler
  Selector : Selector  InputPortWidth=3  IndexOptions=Index vector (dialog)  Indices=3  OutputSizes=1
  Sum : Sum  Inputs=|+-
  Sum2 : Sum  Inputs=|+-
  Wrap Yaw Error : MATLAB Function  TreatAsAtomicUnit=on
  Errors : Outport
  wires:
  EstimatedStates/1 -> Bus Selector2/1
  Reference/1 -> Bus Selector1/1
  Bus Selector1/1 -> Sum/1  "<Position_ref>"
  Bus Selector2/1 -> Sum/2  "<Position>"
  Sum/1 -> Bus Creator/1  "PositionError"
  Bus Selector2/2 -> Selector/1  "<Euler>"
  Bus Selector1/2 -> Sum2/1  "<Yaw_ref>"
  Selector/1 -> Sum2/2  "Yaw_est"
  Sum2/1 -> Wrap Yaw Error/1(YawErrorRaw)  "YawErrorRaw"
  Bus Creator/1 -> Errors/1
  Wrap Yaw Error/1(YawError) -> Bus Creator/2  "YawError"

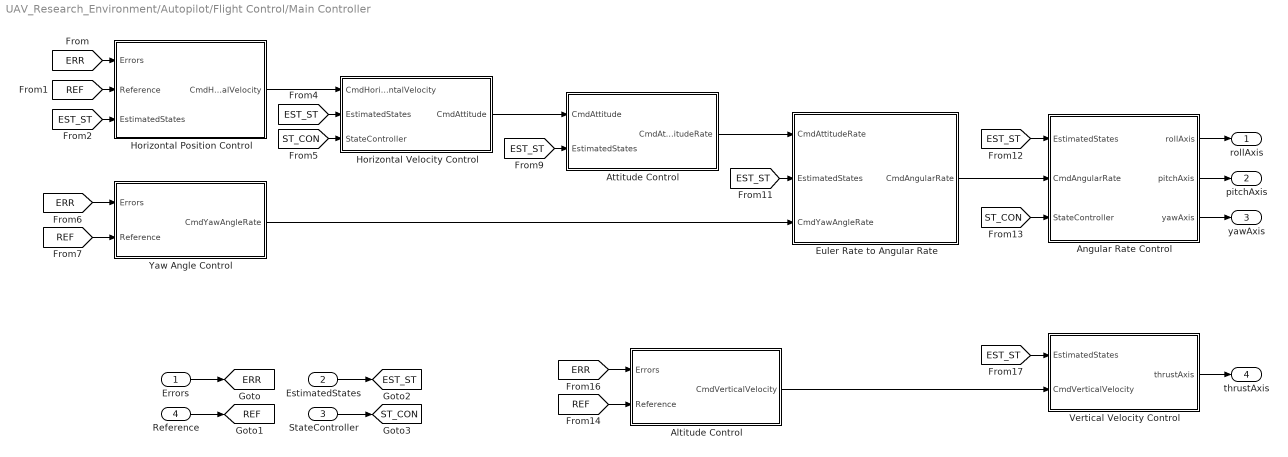
== system UAV_Research_Environment/Autopilot/Flight Control/Main Controller ==
  Errors : Inport
  EstimatedStates : Inport  Port=2
  StateController : Inport  Port=3
  Reference : Inport  Port=4
  Altitude Control : Subsystem
  Angular Rate Control : Subsystem
  Attitude Control : Subsystem
  Euler Rate to Angular Rate : Subsystem
  Horizontal Position Control : Subsystem
  Horizontal Velocity Control : Subsystem
  Vertical Velocity Control : Subsystem
  Yaw Angle Control : Subsystem
  rollAxis : Outport
  pitchAxis : Outport  Port=2
  yawAxis : Outport  Port=3
  thrustAxis : Outport  Port=4
  tag scope: ERR=global, EST_ST=global, REF=global, ST_CON=global
  wires:
  Horizontal Position Control/1(CmdHorizontalVelocity) -> Horizontal Velocity Control/1(CmdHorizontalVelocity)
  Errors/1 -> [ERR]
  Reference/1 -> [REF]
  EstimatedStates/1 -> [EST_ST]
  StateController/1 -> [ST_CON]
  [ERR] -> Horizontal Position Control/1(Errors)
  [REF] -> Horizontal Position Control/2(Reference)
  [EST_ST] -> Horizontal Position Control/3(EstimatedStates)
  [EST_ST] -> Horizontal Velocity Control/2(EstimatedStates)
  [ST_CON] -> Horizontal Velocity Control/3(StateController)
  [ERR] -> Yaw Angle Control/1(Errors)
  [REF] -> Yaw Angle Control/2(Reference)
  Horizontal Velocity Control/1(CmdAttitude) -> Attitude Control/1(CmdAttitude)
  [EST_ST] -> Attitude Control/2(EstimatedStates)
  Attitude Control/1(CmdAttitudeRate) -> Euler Rate to Angular Rate/1(CmdAttitudeRate)
  [EST_ST] -> Euler Rate to Angular Rate/2(EstimatedStates)
  Yaw Angle Control/1(CmdYawAngleRate) -> Euler Rate to Angular Rate/3(CmdYawAngleRate)
  Euler Rate to Angular Rate/1(CmdAngularRate) -> Angular Rate Control/2(CmdAngularRate)
  [ST_CON] -> Angular Rate Control/3(StateController)
  [EST_ST] -> Angular Rate Control/1(EstimatedStates)
  Angular Rate Control/1(rollAxis) -> rollAxis/1
  Angular Rate Control/2(pitchAxis) -> pitchAxis/1
  Angular Rate Control/3(yawAxis) -> yawAxis/1
  [ERR] -> Altitude Control/1(Errors)
  [REF] -> Altitude Control/2(Reference)
  Altitude Control/1(CmdVerticalVelocity) -> Vertical Velocity Control/2(CmdVerticalVelocity)
  [EST_ST] -> Vertical Velocity Control/1(EstimatedStates)
  Vertical Velocity Control/1(thrustAxis) -> thrustAxis/1

== system UAV_Research_Environment/Autopilot/Flight Control/Reference Supervisor ==
  Reference : Inport
  FlightManagement : Inport  Port=2
  EstimatedStates : Inport  Port=3
  Bus Assignment : BusAssignment  AssignedSignals=Position_ref,Velocity_ref,Acceleration_ref,Yaw_ref,YawRate_ref
  Bus Selector : BusSelector  OutputSignals=Position_ref,Velocity_ref,Acceleration_ref,Yaw_ref,YawRate_ref
  Bus Selector1 : BusSelector  OutputSignals=Position,Attitude.Euler
  Bus Selector2 : BusSelector  OutputSignals=mode
  Failsafe_Reference : MATLAB Function  TreatAsAtomicUnit=on
  Rate Transition{,1..4} (5 alike) : RateTransition  OutPortSampleTime=AUTOPILOT.rate.controlSampleTime_s
  descentRate : Constant  Value=AUTOPILOT.failsafe.navigation.descentRate_m_s  SampleTime=AUTOPILOT.rate.controlSampleTime_s
  navFailsafe : Constant  Value=AUTOPILOT.mode.navFailsafe  SampleTime=AUTOPILOT.rate.controlSampleTime_s
  EffectiveReference : Outport
  wires:
  EstimatedStates/1 -> Bus Selector1/1
  FlightManagement/1 -> Bus Selector2/1
  Bus Selector/1 -> Failsafe_Reference/1(Position_ref)  "<Position_ref>"
  Bus Selector/2 -> Failsafe_Reference/2(Velocity_ref)  "<Velocity_ref>"
  Bus Selector/3 -> Failsafe_Reference/3(Acceleration_ref)  "<Acceleration_ref>"
  Bus Selector/4 -> Failsafe_Reference/4(Yaw_ref)  "<Yaw_ref>"
  Bus Selector/5 -> Failsafe_Reference/5(YawRate_ref)  "<YawRate_ref>"
  Bus Selector1/2 -> Failsafe_Reference/7(Euler_est)  "<Euler>"
  Bus Selector1/1 -> Failsafe_Reference/6(Position_est)  "<Position>"
  Bus Selector2/1 -> Failsafe_Reference/8(mode)  "<mode>"
  navFailsafe/1 -> Failsafe_Reference/9(navFailsafe)
  descentRate/1 -> Failsafe_Reference/10(descentRate)
  Failsafe_Reference/1(Position_ref_eff) -> Rate Transition/1
  Failsafe_Reference/2(Velocity_ref_eff) -> Rate Transition1/1
  Failsafe_Reference/3(Acceleration_ref_eff) -> Rate Transition2/1
  Failsafe_Reference/4(Yaw_ref_eff) -> Rate Transition3/1
  Failsafe_Reference/5(YawRate_ref_eff) -> Rate Transition4/1
  Bus Assignment/1 -> EffectiveReference/1
  Rate Transition/1 -> Bus Assignment/2
  Rate Transition1/1 -> Bus Assignment/3
  Rate Transition2/1 -> Bus Assignment/4
  Rate Transition3/1 -> Bus Assignment/5
  Rate Transition4/1 -> Bus Assignment/6
  Reference/1 -> Bus Assignment/1, Bus Selector/1

== system UAV_Research_Environment/Environment/Wind Disturbances/OFF ==
  States : Inport
  Constant : Constant  Value=zeros(3,1)
  Terminator : Terminator
  v_wind : Outport
  w_wind : Outport  Port=2
  wires:
  States/1 -> Terminator/1
  Constant/1 -> w_wind/1, v_wind/1

== system UAV_Research_Environment/Environment/Wind Disturbances/ON ==
  States : Inport
  Bus Selector : BusSelector  OutputSignals=Q
  Bus Selector2 : BusSelector  OutputSignals=Velocity,Position,Attitude
  Constant : Constant  Value=P_ENV.wind.turbulence.speed_epsilon_m_s
  Demux : Demux  Outputs=3
  Dot Product : DotProduct  OutDataTypeStr=Inherit: Inherit via internal rule
  Dryden Wind Turbulence : aerolibwind2/Dryden Wind Turbulence Model  (Continuous (+q -r))  units=Metric (MKS)  spec=MIL-F-8785C  model=Discrete Dryden (+q +r)  W20=P_ENV.wind.turbulence.speed_6m_m_s  Wdeg=P_ENV.wind.turbulence.direction_6m_deg  TurbProb=10^-2 - Light  L_high=P_ENV.wind.turbulence.scale_length_m  Wingspan=P_UAV.geometry.dryden_equivalent_span_m  ts=P_ENV.wind.turbulence.sample_time_s  Seed=P_ENV.wind.turbulence.noise_seeds  T_on=on
      settings: LibrarySourceBlock=|
      | aerolibwind2/Dryden Wind Turbulence Model
      | (Discrete (+q +r))
  Gain : Gain  Gain=-1
  Quaternions to Direction Cosine Matrix : Quat2Dcm
  Sqrt : Sqrt
  Sum : Sum  Inputs=+++
  Sum1 : Sum  Inputs=|++
  Terminator : Terminator
  Terminator1 : Terminator
  Wind Gust : aerolibwind2/Discrete Wind Gust Model  units=Metric (MKS)  Gx=on  Gy=on  Gz=on  t_0=P_ENV.wind.gust.start_time_s  d_m=P_ENV.wind.gust.length_m  v_m=P_ENV.wind.gust.amplitude_m_s
  Wind Shear : aerolibwind2/Wind Shear Model  units=Metric (MKS)  phase=Category C - Terminal Flight Phase  W_20=P_ENV.wind.shear.speed_6m_m_s  Wdeg=P_ENV.wind.shear.direction_6m_deg
  v_wind : Outport
  w_wind : Outport  Port=2
  wires:
  Sum1/1 -> Dryden Wind Turbulence/2
  Dryden Wind Turbulence/1 -> Sum/3
  Gain/1 -> Dryden Wind Turbulence/1, Wind Shear/1
  Constant/1 -> Sum1/2
  Bus Selector2/2 -> Demux/1  "<Position>"
  Bus Selector/1 -> Quaternions to Direction Cosine Matrix/1  "<Q>"
  Sqrt/1 -> Wind Gust/1, Sum1/1
  Bus Selector2/1 -> Dot Product/2, Dot Product/1  "<Velocity>"
  Demux/3 -> Gain/1  "z"
  Quaternions to Direction Cosine Matrix/1 -> Dryden Wind Turbulence/3, Wind Shear/2
  Wind Shear/1 -> Sum/2
  States/1 -> Bus Selector2/1
  Dryden Wind Turbulence/2 -> w_wind/1
  Bus Selector2/3 -> Bus Selector/1  "<Attitude>"
  Wind Gust/1 -> Sum/1
  Dot Product/1 -> Sqrt/1
  Sum/1 -> v_wind/1
  Demux/1 -> Terminator/1
  Demux/2 -> Terminator1/1

== system UAV_Research_Environment/UAV Plant/UAV Analytical [ODEs]/Attitude Kinematics ==
  Omega_body : Inport
  Normalize Quaternion : MATLAB Function  TreatAsAtomicUnit=on
  Quaternion Integrator : Integrator  InitialCondition=A_UAV.init.quaternion_wxyz
  Quaternion Kinematics : MATLAB Function  TreatAsAtomicUnit=on
  Quaternions to Direction Cosine Matrix : Quat2Dcm
  Quaternions to Rotation Angles : Quat2Angle
      settings: AttributesFormatString=Rotation Order: %<rotationOrder>
  Selector : Selector  InputPortWidth=3  IndexOptions=Index vector (dialog)  Indices=[3 2 1]  OutputSizes=1
  Transpose : Math  Operator=transpose
  Euler : Outport
  Q : Outport  Port=2
  R_BN : Outport  Port=3
  wires:
  Omega_body/1 -> Quaternion Kinematics/1(Omega_body)
  Quaternion Integrator/1 -> Normalize Quaternion/1(Q_raw)
  Quaternion Kinematics/1(Q_dot) -> Quaternion Integrator/1
  Normalize Quaternion/1(Q) -> Quaternions to Rotation Angles/1, Quaternions to Direction Cosine Matrix/1, Q/1, Quaternion Kinematics/2(Q)
  Quaternions to Rotation Angles/1 -> Selector/1
  Selector/1 -> Euler/1
  Quaternions to Direction Cosine Matrix/1 -> Transpose/1
  Transpose/1 -> R_BN/1

== system UAV_Research_Environment/UAV Plant/UAV Analytical [ODEs]/Ground Contact ==
  p_ned : Inport
  v_ned : Inport  Port=2
  R_BN : Inport  Port=3
  Omega_body : Inport  Port=4
  Ground_Contact_Model : MATLAB Function  TreatAsAtomicUnit=on
  F_ground_body : Outport
  Tau_ground_body : Outport  Port=2
  wires:
  p_ned/1 -> Ground_Contact_Model/1(p_ned)
  v_ned/1 -> Ground_Contact_Model/2(v_ned)
  R_BN/1 -> Ground_Contact_Model/3(R_BN)
  Omega_body/1 -> Ground_Contact_Model/4(Omega_body)
  Ground_Contact_Model/1(F_ground_body) -> F_ground_body/1
  Ground_Contact_Model/2(Tau_ground_body) -> Tau_ground_body/1

== system UAV_Research_Environment/UAV Plant/UAV Analytical [ODEs]/Pitch Moment ==
  T : Inport
  Demux : Demux
  Gain : Gain  Gain=A_UAV.rotor.arm_body_m(1,1)
  Gain1 : Gain  Gain=A_UAV.rotor.arm_body_m(2,1)
  Gain2 : Gain  Gain=A_UAV.rotor.arm_body_m(3,1)
  Gain3 : Gain  Gain=A_UAV.rotor.arm_body_m(4,1)
  Sum : Sum  Inputs=++++
  Tau_y : Outport
  wires:
  T/1 -> Demux/1
  Demux/1 -> Gain/1
  Demux/2 -> Gain1/1
  Demux/3 -> Gain2/1
  Demux/4 -> Gain3/1
  Gain/1 -> Sum/1
  Gain1/1 -> Sum/2
  Gain2/1 -> Sum/3
  Gain3/1 -> Sum/4
  Sum/1 -> Tau_y/1  "Tau_y"

== system UAV_Research_Environment/UAV Plant/UAV Analytical [ODEs]/Roll Moment ==
  T : Inport
  Demux : Demux
  Gain : Gain  Gain=-A_UAV.rotor.arm_body_m(1,2)
  Gain1 : Gain  Gain=-A_UAV.rotor.arm_body_m(2,2)
  Gain2 : Gain  Gain=-A_UAV.rotor.arm_body_m(3,2)
  Gain3 : Gain  Gain=-A_UAV.rotor.arm_body_m(4,2)
  Sum : Sum  Inputs=++++
  Tau_x : Outport
  wires:
  T/1 -> Demux/1
  Demux/1 -> Gain/1
  Demux/2 -> Gain1/1
  Demux/3 -> Gain2/1
  Demux/4 -> Gain3/1
  Gain/1 -> Sum/1
  Gain1/1 -> Sum/2
  Gain2/1 -> Sum/3
  Gain3/1 -> Sum/4
  Sum/1 -> Tau_x/1  "Tau_x"

== system UAV_Research_Environment/UAV Plant/UAV Analytical [ODEs]/Rotational Dynamics ==
  "Tau_body " : Inport
  Wind_w : Inport  Port=2
  Body Angular Rate : Integrator  InitialCondition=A_UAV.init.body_rate_rad_s
  Constant : Constant  Value=A_UAV.aero.angular_damping_Nm_per_rad_s
  Gain : Gain  Gain=-1
  Gyroscopic Term : Subsystem
  Inertia Matrix : Gain  Gain=A_UAV.rigid.inertia_kgm2  Multiplication=Matrix(K*u)
  Inverse Inertia : Gain  Gain=A_UAV.rigid.inertia_inverse_1_kgm2  Multiplication=Matrix(K*u)
  Product : Product
  Sum : Sum  Inputs=-++
  Sum1 : Sum  Inputs=|+-
  Omega_body : Outport
  wires:
  Body Angular Rate/1 -> Omega_body/1, Sum1/1, Gyroscopic Term/1("Omega_body "), Inertia Matrix/1  "Omega_body"
  Inertia Matrix/1 -> Gyroscopic Term/2("I_Omega    ")  "I_omega"
  Sum/1 -> Inverse Inertia/1
  Inverse Inertia/1 -> Body Angular Rate/1
  Wind_w/1 -> Sum1/2
  Sum1/1 -> Product/1  "Omega_rel_body"
  Product/1 -> Gain/1
  Constant/1 -> Product/2
  Gain/1 -> Sum/3  "Tau_aero_body"
  "Tau_body "/1 -> Sum/2
  Gyroscopic Term/1(Gyro) -> Sum/1

== system UAV_Research_Environment/UAV Plant/UAV Analytical [ODEs]/Rotor Force ==
  T : Inport
  Demux : Demux
  "Fx, Fy" : Constant  Value=0
  Gain : Gain  Gain=-1
  Mux : Mux  Inputs=3
  Sum : Sum  Inputs=++++
  F_body : Outport
  wires:
  T/1 -> Demux/1
  Demux/1 -> Sum/1
  Demux/2 -> Sum/2
  Demux/3 -> Sum/3
  Demux/4 -> Sum/4
  Sum/1 -> Gain/1  "T_R"
  "Fx, Fy"/1 -> Mux/1, Mux/2
  Mux/1 -> F_body/1  "F_body"
  Gain/1 -> Mux/3  "Fz"

== system UAV_Research_Environment/UAV Plant/UAV Analytical [ODEs]/Rotor Reaction Torque ==
  Omega : Inport
  C_Q : Gain  Gain=A_UAV.rotor.cQ_Nm_per_rad_s_sq
  Product : Product
  Q : Outport
  wires:
  Omega/1 -> Product/1, Product/2
  Product/1 -> C_Q/1  "Omega_sq"
  C_Q/1 -> Q/1  "Q"

== system UAV_Research_Environment/UAV Plant/UAV Analytical [ODEs]/Rotor Thrust ==
  Omega : Inport
  C_T : Gain  Gain=A_UAV.rotor.cT_N_per_rad_s_sq
  Product : Product
  T : Outport
  wires:
  Omega/1 -> Product/1, Product/2
  Product/1 -> C_T/1  "Omega_sq"
  C_T/1 -> T/1  "T"

== system UAV_Research_Environment/UAV Plant/UAV Analytical [ODEs]/State Outputs ==
  v_ned : Inport
  p_ned : Inport  Port=2
  a_ned : Inport  Port=3
  Euler : Inport  Port=4
  Q : Inport  Port=5
  Omega_body : Inport  Port=6
  Bus Creator : BusCreator  Inputs=5
  Bus Creator1 : BusCreator  Inputs=2
  States : Outport
  wires:
  Bus Creator/1 -> States/1
  p_ned/1 -> Bus Creator/1  "Position"
  v_ned/1 -> Bus Creator/2  "Velocity"
  a_ned/1 -> Bus Creator/3  "Acceleration"
  Omega_body/1 -> Bus Creator/4  "AngularRate"
  Bus Creator1/1 -> Bus Creator/5  "Attitude"
  Q/1 -> Bus Creator1/1  "Q"
  Euler/1 -> Bus Creator1/2  "Euler"

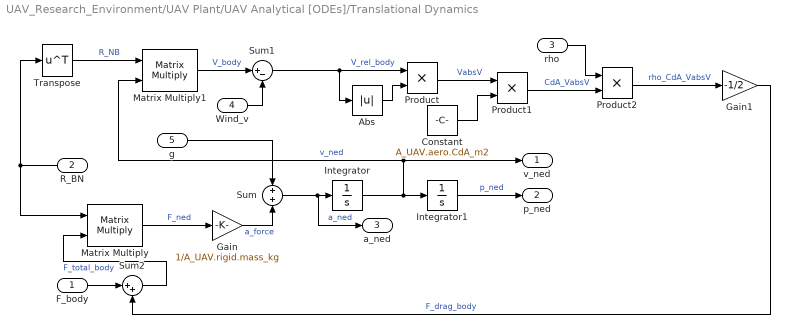
== system UAV_Research_Environment/UAV Plant/UAV Analytical [ODEs]/Translational Dynamics ==
  F_body : Inport
  R_BN : Inport  Port=2
  rho : Inport  Port=3
  Wind_v : Inport  Port=4
  g : Inport  Port=5
  Abs : Abs  SaturateOnIntegerOverflow=off
  Constant : Constant  Value=A_UAV.aero.CdA_m2
  Gain : Gain  Gain=1/A_UAV.rigid.mass_kg
  Gain1 : Gain  Gain=-1/2
  Integrator : Integrator  InitialCondition=A_UAV.init.velocity_ned_m_s
  Integrator1 : Integrator  InitialCondition=A_UAV.init.position_ned_m
  Matrix Multiply : Product  Multiplication=Matrix(*)
  Matrix Multiply1 : Product  Multiplication=Matrix(*)
  Product : Product
  Product1 : Product
  Product2 : Product
  Sum : Sum
  Sum1 : Sum  Inputs=|+-
  Sum2 : Sum  Inputs=|++
  Transpose : Math  Operator=transpose
  v_ned : Outport
  p_ned : Outport  Port=2
  a_ned : Outport  Port=3
  wires:
  Matrix Multiply/1 -> Gain/1  "F_ned"
  Gain/1 -> Sum/2  "a_force"
  Sum/1 -> a_ned/1, Integrator/1  "a_ned"
  Integrator/1 -> Matrix Multiply1/2, v_ned/1, Integrator1/1  "v_ned"
  Integrator1/1 -> p_ned/1  "p_ned"
  R_BN/1 -> Matrix Multiply/1, Transpose/1
  g/1 -> Sum/1
  Transpose/1 -> Matrix Multiply1/1  "R_NB"
  Matrix Multiply1/1 -> Sum1/1  "V_body"
  Wind_v/1 -> Sum1/2
  Sum1/1 -> Product/1, Abs/1  "V_rel_body"
  Abs/1 -> Product/2
  Product/1 -> Product1/1  "VabsV"
  Constant/1 -> Product1/2
  Product1/1 -> Product2/2  "CdA_VabsV"
  rho/1 -> Product2/1
  Product2/1 -> Gain1/1  "rho_CdA_VabsV"
  Gain1/1 -> Sum2/2  "F_drag_body"
  F_body/1 -> Sum2/1
  Sum2/1 -> Matrix Multiply/2  "F_total_body"

== system UAV_Research_Environment/UAV Plant/UAV Analytical [ODEs]/Yaw Moment ==
  Q : Inport
  Demux : Demux
  Gain : Gain  Gain=A_UAV.rotor.spin_direction(1)
  Gain1 : Gain  Gain=A_UAV.rotor.spin_direction(2)
  Gain2 : Gain  Gain=A_UAV.rotor.spin_direction(3)
  Gain3 : Gain  Gain=A_UAV.rotor.spin_direction(4)
  Sum : Sum  Inputs=++++
  Tau_z : Outport
  wires:
  Q/1 -> Demux/1
  Demux/1 -> Gain/1
  Demux/2 -> Gain1/1
  Demux/3 -> Gain2/1
  Demux/4 -> Gain3/1
  Gain/1 -> Sum/1
  Gain1/1 -> Sum/2
  Gain2/1 -> Sum/3
  Gain3/1 -> Sum/4
  Sum/1 -> Tau_z/1  "Tau_z"

== system UAV_Research_Environment/UAV Plant/UAV Block [Simulink Blocks]/State Outputs ==
  Ve : Inport
  Xe : Inport  Port=2
  Angles : Inport  Port=3
  Q : Inport  Port=4
  wb : Inport  Port=5
  a_ned : Inport  Port=6
  Bus Creator : BusCreator  Inputs=2
  Bus Creator1 : BusCreator  Inputs=5
  States : Outport
  wires:
  Xe/1 -> Bus Creator1/1  "Position"
  Ve/1 -> Bus Creator1/2  "Velocity"
  a_ned/1 -> Bus Creator1/3  "Acceleration"
  wb/1 -> Bus Creator1/4  "AngularRate"
  Bus Creator/1 -> Bus Creator1/5  "Attitude"
  Angles/1 -> Bus Creator/2  "Euler"
  Q/1 -> Bus Creator/1  "Q"
  Bus Creator1/1 -> States/1
